simulink model "UNO_Generic_task"  (Simulink 3.00)
undefined symbols (not defined in the file): Double, F64
libraries: mathlib x7, REXduino_library x5, arclib x2, genlib x1

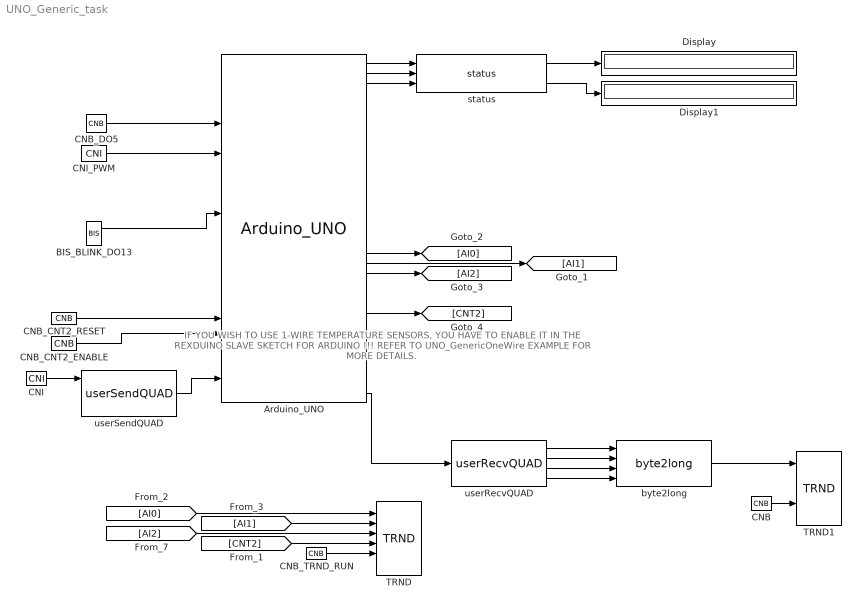
== system UNO_Generic_task ==
  note: IF YOU WISH TO USE 1-WIRE TEMPERATURE SENSORS,
      | YOU HAVE TO ENABLE IT IN THE REXDUINO SLAVE SKETCH
      | FOR ARDUINO !!!
      |
      | REFER TO UNO_GenericOneWire EXAMPLE FOR MORE DETAILS.
  Arduino_UNO : REXduino_library/Arduino_UNO  comPort=COM3  pinmode2=8: Counter  pinmode3=1: Not connected  pinmode4=10: Counter DIR / Encoder B  pinmode5=2: Digital output  pinmode6=1: Not connected  pinmode9=5: PWM (analog output)  pinmode10=1: Not connected  pinmode11=1: Not connected  pinmodeA0=6: Analog input  pinmodeA1=6: Analog input  pinmodeA2=6: Analog input  pinmodeA3=1: Not connected  pinmodeA4=1: Not connected  pinmodeA5=1: Not connected  usercmd=2: Four bytes
  BIS_BLINK_DO13 : genlib/BIS  Y0=off  t1=0.7  t2=0.8  t3=0.9  t4=1  t5=0  t6=6  t7=7  t8=8  RPT=on  bEdit=off
  CNB : mathlib/CNB  YCN=on
  CNB_CNT2_ENABLE : mathlib/CNB  YCN=on
  CNB_CNT2_RESET : mathlib/CNB  YCN=off
  CNB_DO5 : mathlib/CNB  YCN=on
  CNB_TRND_RUN : mathlib/CNB  YCN=on
  CNI : mathlib/CNI  icn=1
  CNI_PWM : mathlib/CNI  icn=128
  Display : Display
      settings: Format=Best fit
  Display1 : Display
      settings: Format=Best fit
  TRND : arclib/TRND  n=4  l=1000  btype=8: Double  ptype1=1: Store  ptype2=1: Store  ptype3=1: Store  ptype4=1: Store  pfac=1  afac=0  arc=0  id=1  Title=Data trend  timesrc=1
  TRND1 : arclib/TRND  n=4  l=1000  btype=8: Double (F64)  ptype1=1: Store  ptype2=1: Store  ptype3=1: Store  ptype4=1: Store  pfac=1  afac=0  arc=0  id=0  Title=Trend Title  timesrc=1: CORETIMER
  byte2long : REXduino_library/byte2long
      mask Type: REX sequence
  status : REXduino_library/status
      mask Type: REX sequence
  userRecvQUAD : REXduino_library/userRecvQUAD
      mask Type: REX sequence
  userSendQUAD : REXduino_library/userSendQUAD
      mask Type: REX sequence
  wires:
  Arduino_UNO/1 -> status/1
  Arduino_UNO/2 -> status/2
  Arduino_UNO/3 -> status/3
  Arduino_UNO/20 -> [AI0]
  Arduino_UNO/21 -> [AI1]
  Arduino_UNO/22 -> [AI2]
  Arduino_UNO/26 -> [CNT2]
  Arduino_UNO/34 -> userRecvQUAD/1
  BIS_BLINK_DO13/1 -> Arduino_UNO/10
  CNB/1 -> TRND1/5
  CNB_CNT2_ENABLE/1 -> Arduino_UNO/18
  CNB_CNT2_RESET/1 -> Arduino_UNO/17
  CNB_DO5/1 -> Arduino_UNO/4
  CNB_TRND_RUN/1 -> TRND/5
  CNI/1 -> userSendQUAD/1
  CNI_PWM/1 -> Arduino_UNO/6
  [CNT2] -> TRND/4
  [AI0] -> TRND/1
  [AI1] -> TRND/2
  [AI2] -> TRND/3
  byte2long/1 -> TRND1/1
  status/1 -> Display/1
  status/2 -> Display1/1
  userRecvQUAD/1 -> byte2long/1
  userRecvQUAD/2 -> byte2long/2
  userRecvQUAD/3 -> byte2long/3
  userRecvQUAD/4 -> byte2long/4
  userSendQUAD/1 -> Arduino_UNO/21
